simulink model "filter_bank"  (R2020b)
settings: Solver=FixedStepDiscrete  StartTime=0.0  StopTime=0.01  FixedStep=1.6276041666666666e-07  RelTol=1e-3
undefined symbols (not defined in the file or in its folder): mp
libraries: hdlsllib x2, simulink x1
settings Model: DataTypeOverride=Off  Creator=Ross  LastModifiedBy=conno
settings DataIOCC: SaveOutput=off  SaveTime=off  ReturnWorkspaceOutputs=off
settings OptimizationCC: BlockReduction=off  ConditionallyExecuteInputs=off  DefaultParameterBehavior=Inlined
settings DebuggingCC: ReadBeforeWriteMsg=DisableAll  WriteAfterWriteMsg=DisableAll  WriteAfterReadMsg=DisableAll  AlgebraicLoopMsg=error  MultiTaskDSMMsg=none  SingleTaskRateTransMsg=error  PregeneratedLibrarySubsystemCodeDiagnostic=none  ArithmeticOperatorsInVariantConditions=warning
settings HardwareCC: ProdBitPerPointer=32  ProdBitPerSizeT=32  ProdBitPerPtrDiffT=32  ProdLargestAtomicFloat=None  ProdIntDivRoundTo=Undefined  ProdEndianess=Unspecified  ProdWordSize=32  ProdHWDeviceType=ASIC/FPGA->ASIC/FPGA  TargetBitPerPointer=64  TargetBitPerSizeT=64  TargetBitPerPtrDiffT=64  TargetLongLongMode=on  TargetIntDivRoundTo=Zero  TargetEndianess=LittleEndian  TargetWordSize=64  TargetHWDeviceType=Custom Processor->MATLAB Host Computer  ProdEqTarget=off
settings ModelReferenceCC: UpdateModelReferenceTargets=IfOutOfDate
settings SFSimCC: SFSimEcho=off  SimUseLocalCustomCode=off  CustomCodeUndefinedFunction=UseInterfaceOnly
settings RTWCC: RTWUseLocalCustomCode=off

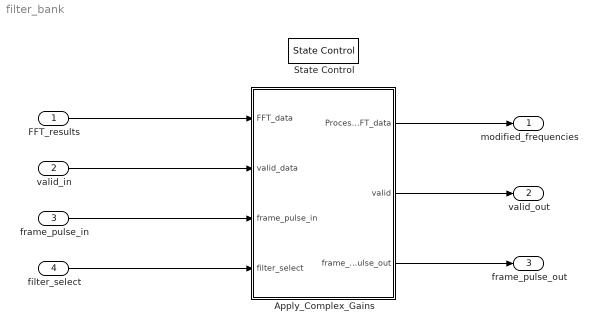
== system filter_bank ==
  FFT_results : Inport  OutDataTypeStr=fixdt(1,31,23)  PortDimensions=1  SampleTime=[1.6276041666666666e-07,0]
      settings: SignalType=complex
  valid_in : Inport  Port=2  OutDataTypeStr=boolean  PortDimensions=1  SampleTime=[1.6276041666666666e-07,0]
  frame_pulse_in : Inport  Port=3  OutDataTypeStr=boolean  PortDimensions=1  SampleTime=[1.6276041666666666e-07,0]
  filter_select : Inport  Port=4  OutDataTypeStr=fixdt(0,2,0)  PortDimensions=1  SampleTime=[1.6276041666666666e-07,0]
  Apply_Complex_Gains : Subsystem
  State Control : StateControl  StateControl=Synchronous
  modified_frequencies : Outport  PortDimensions=1  SampleTime=[1.6276041666666666e-07,0]  VectorParamsAs1DForOutWhenUnconnected=off
      settings: SignalType=complex
  valid_out : Outport  Port=2  OutDataTypeStr=boolean  PortDimensions=1  SampleTime=[1.6276041666666666e-07,0]  VectorParamsAs1DForOutWhenUnconnected=off
  frame_pulse_out : Outport  Port=3  OutDataTypeStr=boolean  PortDimensions=1  SampleTime=[1.6276041666666666e-07,0]
  wires:
  FFT_results/1 -> Apply_Complex_Gains/1(FFT_data)
  valid_in/1 -> Apply_Complex_Gains/2(valid_data)
  frame_pulse_in/1 -> Apply_Complex_Gains/3(frame_pulse_in)
  Apply_Complex_Gains/1(Processed_FFT_data) -> modified_frequencies/1
  Apply_Complex_Gains/2(valid) -> valid_out/1
  Apply_Complex_Gains/3(frame_pulse_out) -> frame_pulse_out/1
  filter_select/1 -> Apply_Complex_Gains/4(filter_select)

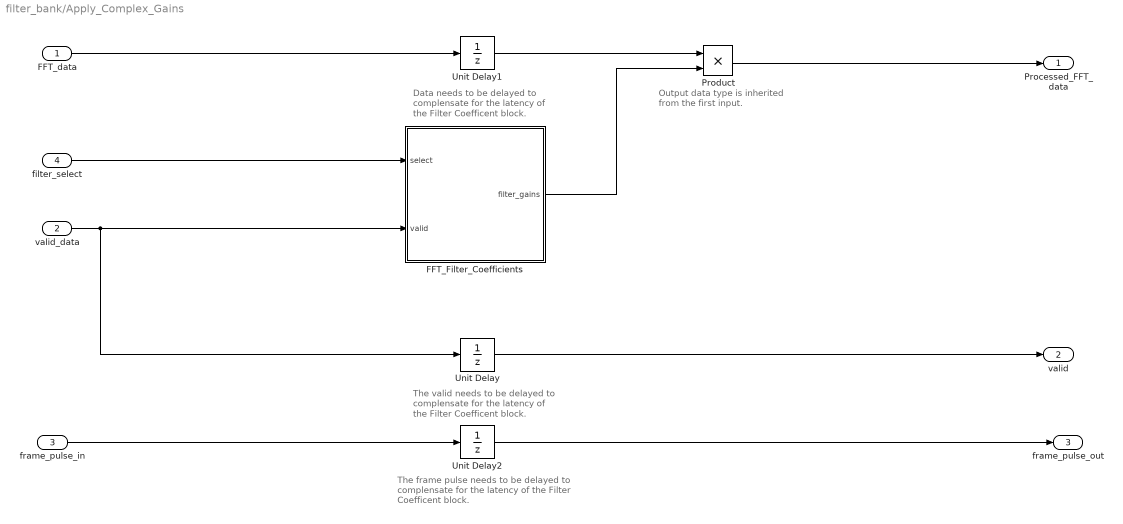
== system filter_bank/Apply_Complex_Gains ==
  note: Data needs to be delayed
      | to complensate for the latency
      | of the Filter Coefficent block.
  note: The valid needs to be delayed
      | to complensate for the latency
      | of the Filter Coefficent block.
  note: The frame pulse needs to be delayed
      | to complensate for the latency
      | of the Filter Coefficent block.
  note: Output data type is inherited
      | from the first input.
  FFT_data : Inport
  valid_data : Inport  Port=2
  frame_pulse_in : Inport  Port=3
  filter_select : Inport  Port=4
  FFT_Filter_Coefficients : Subsystem
  Product : Product  OutDataTypeStr=Inherit: Same as first input
  Unit Delay : UnitDelay  SampleTime=-1  HasFrameUpgradeWarning=on
  Unit Delay1 : UnitDelay  SampleTime=-1  HasFrameUpgradeWarning=on
  Unit Delay2 : UnitDelay  SampleTime=-1  HasFrameUpgradeWarning=on
  Processed_FFT_data : Outport
  valid : Outport  Port=2
  frame_pulse_out : Outport  Port=3
  wires:
  Unit Delay1/1 -> Product/1
  Unit Delay/1 -> valid/1
  Product/1 -> Processed_FFT_data/1
  FFT_Filter_Coefficients/1(filter_gains) -> Product/2
  filter_select/1 -> FFT_Filter_Coefficients/1(select)
  Unit Delay2/1 -> frame_pulse_out/1
  frame_pulse_in/1 -> Unit Delay2/1
  FFT_data/1 -> Unit Delay1/1
  valid_data/1 -> FFT_Filter_Coefficients/2(valid), Unit Delay/1

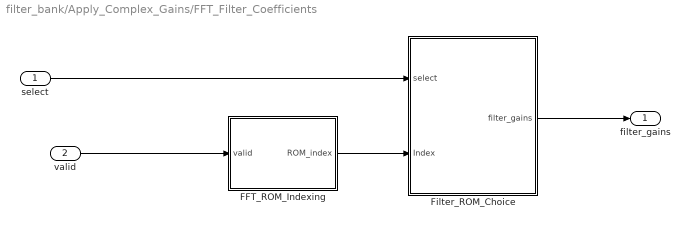
== system filter_bank/Apply_Complex_Gains/FFT_Filter_Coefficients ==
  select : Inport
  valid : Inport  Port=2
  FFT_ROM_Indexing : Subsystem
  Filter_ROM_Choice : Subsystem
  filter_gains : Outport
  wires:
  Filter_ROM_Choice/1(filter_gains) -> filter_gains/1
  select/1 -> Filter_ROM_Choice/1(select)
  valid/1 -> FFT_ROM_Indexing/1(valid)
  FFT_ROM_Indexing/1(ROM_index) -> Filter_ROM_Choice/2(Index)

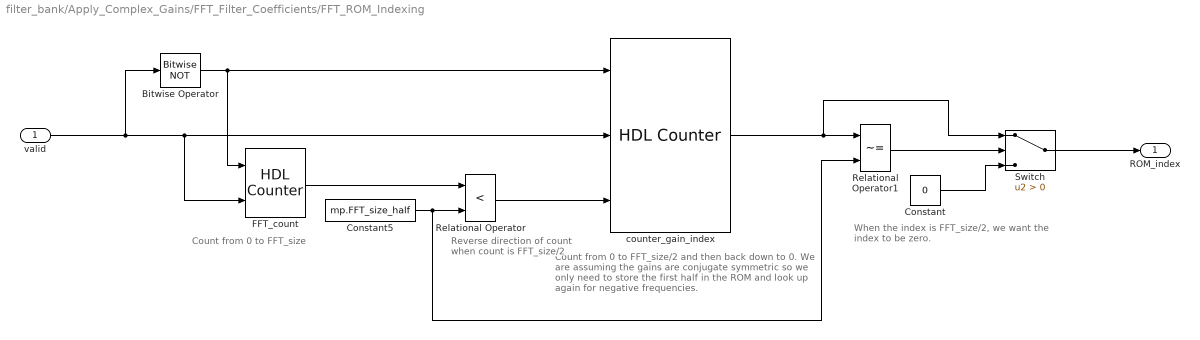
== system filter_bank/Apply_Complex_Gains/FFT_Filter_Coefficients/FFT_ROM_Indexing ==
  note: Count from 0 to FFT_size/2 and then back down to 0.
      | We are assuming the gains are conjugate symmetric
      | so we only need to store the first half in the ROM
      | and look up again for negative frequencies.
  note: Reverse direction of
      | count when count
      | is FFT_size/2
  note: Count from 0 to FFT_size
  note: When the index is FFT_size/2, we want the
      | index to be zero.
  valid : Inport
  Bitwise Operator : simulink/Logic and Bit Operations/Bitwise Operator  logicop=NOT  UseBitMask=off  BitMask=bin2dec('11011001')  BitMaskRealWorld=Stored Integer
  Constant : Constant  Value=0  OutDataTypeStr=fixdt(0,mp.FFT_size_Nbits,0)  SampleTime=mp.Ts/mp.SysRate_Upsample_Factor
  Constant5 : Constant  Value=mp.FFT_size_half  OutDataTypeStr=fixdt(0,mp.FFT_size_Nbits,0)  SampleTime=mp.Ts/mp.SysRate_Upsample_Factor
  FFT_count : hdlsllib/Sources/HDL Counter  CountType=Free running  CountInit=0  CountStep=1  CountMax=25  CountFromType=Initial value  CountFrom=0  CountResetPort=on  CountLoadPort=off  CountEnbPort=on  CountDirPort=off  CountDataType=Unsigned  CountWordLen=mp.FFT_size_Nbits  CountFracLen=0  CountSampTime=1
  Relational Operator : RelationalOperator  Operator=<  OutDataTypeStr=boolean  ZeroCross=off  RndMeth=Nearest
  Relational Operator1 : RelationalOperator  Operator=~=  OutDataTypeStr=boolean  ZeroCross=off  RndMeth=Nearest
  Switch : Switch  Criteria=u2 > Threshold
  counter_gain_index : hdlsllib/Sources/HDL Counter  CountType=Free running  CountInit=0  CountStep=1  CountMax=25  CountFromType=Initial value  CountFrom=0  CountResetPort=on  CountLoadPort=off  CountEnbPort=on  CountDirPort=on  CountDataType=Unsigned  CountWordLen=mp.FFT_size_Nbits  CountFracLen=0  CountSampTime=1
  ROM_index : Outport
  wires:
  Switch/1 -> ROM_index/1
  Constant/1 -> Switch/3
  counter_gain_index/1 -> Relational Operator1/1, Switch/1
  Constant5/1 -> Relational Operator/2, Relational Operator1/2
  valid/1 -> Bitwise Operator/1, counter_gain_index/2, FFT_count/2
  FFT_count/1 -> Relational Operator/1
  Relational Operator1/1 -> Switch/2
  Bitwise Operator/1 -> counter_gain_index/1, FFT_count/1
  Relational Operator/1 -> counter_gain_index/3

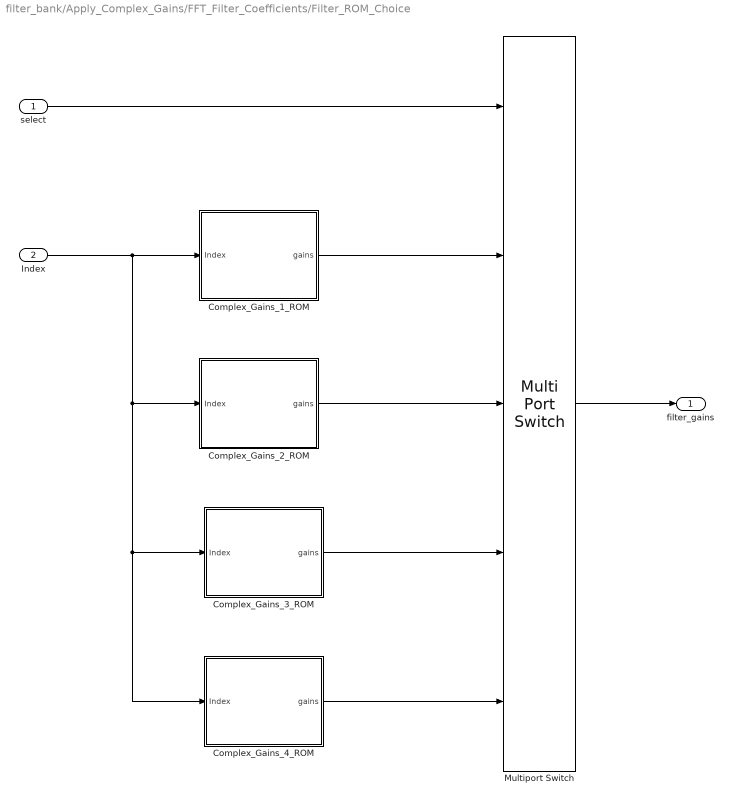
== system filter_bank/Apply_Complex_Gains/FFT_Filter_Coefficients/Filter_ROM_Choice ==
  select : Inport
  Index : Inport  Port=2
  Complex_Gains_1_ROM : Subsystem
  Complex_Gains_2_ROM : Subsystem
  Complex_Gains_3_ROM : Subsystem
  Complex_Gains_4_ROM : Subsystem
  Multiport Switch : MultiPortSwitch  DataPortOrder=Zero-based contiguous  Inputs=4  zeroidx=on
  filter_gains : Outport
  wires:
  Complex_Gains_3_ROM/1(gains) -> Multiport Switch/4
  select/1 -> Multiport Switch/1
  Complex_Gains_2_ROM/1(gains) -> Multiport Switch/3
  Complex_Gains_1_ROM/1(gains) -> Multiport Switch/2
  Complex_Gains_4_ROM/1(gains) -> Multiport Switch/5
  Index/1 -> Complex_Gains_4_ROM/1(Index), Complex_Gains_3_ROM/1(Index), Complex_Gains_2_ROM/1(Index), Complex_Gains_1_ROM/1(Index)
  Multiport Switch/1 -> filter_gains/1

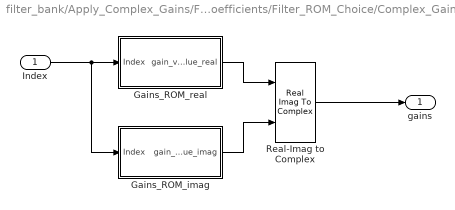
== system filter_bank/Apply_Complex_Gains/FFT_Filter_Coefficients/Filter_ROM_Choice/Complex_Gains_1_ROM ==
  Index : Inport
  Gains_ROM_imag : Subsystem
  Gains_ROM_real : Subsystem
  Real-Imag to Complex : RealImagToComplex
  gains : Outport
  wires:
  Real-Imag to Complex/1 -> gains/1
  Gains_ROM_real/1(gain_value_real) -> Real-Imag to Complex/1
  Index/1 -> Gains_ROM_real/1(Index), Gains_ROM_imag/1(Index)
  Gains_ROM_imag/1(gain_value_imag) -> Real-Imag to Complex/2

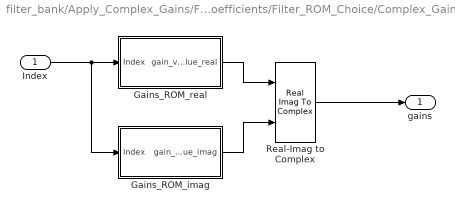
== system filter_bank/Apply_Complex_Gains/FFT_Filter_Coefficients/Filter_ROM_Choice/Complex_Gains_2_ROM ==
  Index : Inport
  Gains_ROM_imag : Subsystem
  Gains_ROM_real : Subsystem
  Real-Imag to Complex : RealImagToComplex
  gains : Outport
  wires:
  Real-Imag to Complex/1 -> gains/1
  Gains_ROM_real/1(gain_value_real) -> Real-Imag to Complex/1
  Index/1 -> Gains_ROM_real/1(Index), Gains_ROM_imag/1(Index)
  Gains_ROM_imag/1(gain_value_imag) -> Real-Imag to Complex/2

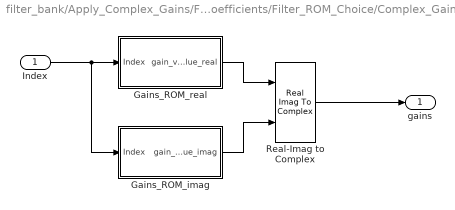
== system filter_bank/Apply_Complex_Gains/FFT_Filter_Coefficients/Filter_ROM_Choice/Complex_Gains_3_ROM ==
  Index : Inport
  Gains_ROM_imag : Subsystem
  Gains_ROM_real : Subsystem
  Real-Imag to Complex : RealImagToComplex
  gains : Outport
  wires:
  Real-Imag to Complex/1 -> gains/1
  Gains_ROM_real/1(gain_value_real) -> Real-Imag to Complex/1
  Index/1 -> Gains_ROM_real/1(Index), Gains_ROM_imag/1(Index)
  Gains_ROM_imag/1(gain_value_imag) -> Real-Imag to Complex/2

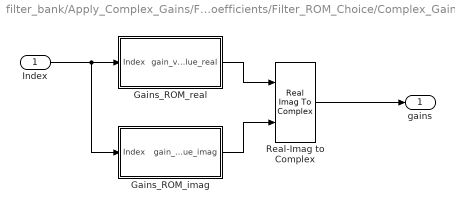
== system filter_bank/Apply_Complex_Gains/FFT_Filter_Coefficients/Filter_ROM_Choice/Complex_Gains_4_ROM ==
  Index : Inport
  Gains_ROM_imag : Subsystem
  Gains_ROM_real : Subsystem
  Real-Imag to Complex : RealImagToComplex
  gains : Outport
  wires:
  Real-Imag to Complex/1 -> gains/1
  Gains_ROM_real/1(gain_value_real) -> Real-Imag to Complex/1
  Index/1 -> Gains_ROM_real/1(Index), Gains_ROM_imag/1(Index)
  Gains_ROM_imag/1(gain_value_imag) -> Real-Imag to Complex/2

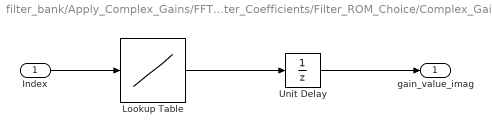
== system filter_bank/Apply_Complex_Gains/FFT_Filter_Coefficients/Filter_ROM_Choice/Complex_Gains_1_ROM/Gains_ROM_imag ==
  Index : Inport
  Lookup Table : Lookup_n-D  NumberOfTableDimensions=1  BreakpointsForDimension1=[0:mp.FFT_size_half-1]  IndexSearchMethod=Evenly spaced points  Table=mp.fft_gains_1_imag  InterpMethod=Flat  ExtrapMethod=Clip  DiagnosticForOutOfRangeInput=Error  UseLastTableValue=on  OutDataTypeStr=fixdt(1,mp.W_bits,mp.F_bits)  RndMeth=Simplest  InputSameDT=on
  Unit Delay : UnitDelay  SampleTime=-1  HasFrameUpgradeWarning=on
  gain_value_imag : Outport  VectorParamsAs1DForOutWhenUnconnected=off
  wires:
  Lookup Table/1 -> Unit Delay/1
  Index/1 -> Lookup Table/1
  Unit Delay/1 -> gain_value_imag/1

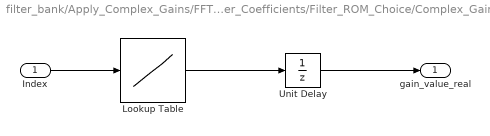
== system filter_bank/Apply_Complex_Gains/FFT_Filter_Coefficients/Filter_ROM_Choice/Complex_Gains_1_ROM/Gains_ROM_real ==
  Index : Inport
  Lookup Table : Lookup_n-D  NumberOfTableDimensions=1  BreakpointsForDimension1=[0:mp.FFT_size_half-1]  IndexSearchMethod=Evenly spaced points  Table=mp.fft_gains_1_real  InterpMethod=Flat  ExtrapMethod=Clip  DiagnosticForOutOfRangeInput=Error  UseLastTableValue=on  OutDataTypeStr=fixdt(1,mp.W_bits,mp.F_bits)  RndMeth=Simplest  InputSameDT=on
  Unit Delay : UnitDelay  SampleTime=-1  HasFrameUpgradeWarning=on
  gain_value_real : Outport  VectorParamsAs1DForOutWhenUnconnected=off
  wires:
  Lookup Table/1 -> Unit Delay/1
  Index/1 -> Lookup Table/1
  Unit Delay/1 -> gain_value_real/1

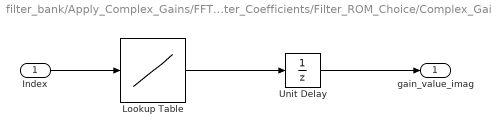
== system filter_bank/Apply_Complex_Gains/FFT_Filter_Coefficients/Filter_ROM_Choice/Complex_Gains_2_ROM/Gains_ROM_imag ==
  Index : Inport
  Lookup Table : Lookup_n-D  NumberOfTableDimensions=1  BreakpointsForDimension1=[0:mp.FFT_size_half-1]  IndexSearchMethod=Evenly spaced points  Table=mp.fft_gains_2_imag  InterpMethod=Flat  ExtrapMethod=Clip  DiagnosticForOutOfRangeInput=Error  UseLastTableValue=on  OutDataTypeStr=fixdt(1,mp.W_bits,mp.F_bits)  RndMeth=Simplest  InputSameDT=on
  Unit Delay : UnitDelay  SampleTime=-1  HasFrameUpgradeWarning=on
  gain_value_imag : Outport  VectorParamsAs1DForOutWhenUnconnected=off
  wires:
  Lookup Table/1 -> Unit Delay/1
  Index/1 -> Lookup Table/1
  Unit Delay/1 -> gain_value_imag/1

== system filter_bank/Apply_Complex_Gains/FFT_Filter_Coefficients/Filter_ROM_Choice/Complex_Gains_2_ROM/Gains_ROM_real ==
  Index : Inport
  Lookup Table : Lookup_n-D  NumberOfTableDimensions=1  BreakpointsForDimension1=[0:mp.FFT_size_half-1]  IndexSearchMethod=Evenly spaced points  Table=mp.fft_gains_2_real  InterpMethod=Flat  ExtrapMethod=Clip  DiagnosticForOutOfRangeInput=Error  UseLastTableValue=on  OutDataTypeStr=fixdt(1,mp.W_bits,mp.F_bits)  RndMeth=Simplest  InputSameDT=on
  Unit Delay : UnitDelay  SampleTime=-1  HasFrameUpgradeWarning=on
  gain_value_real : Outport  VectorParamsAs1DForOutWhenUnconnected=off
  wires:
  Lookup Table/1 -> Unit Delay/1
  Index/1 -> Lookup Table/1
  Unit Delay/1 -> gain_value_real/1

== system filter_bank/Apply_Complex_Gains/FFT_Filter_Coefficients/Filter_ROM_Choice/Complex_Gains_3_ROM/Gains_ROM_imag ==
  Index : Inport
  Lookup Table : Lookup_n-D  NumberOfTableDimensions=1  BreakpointsForDimension1=[0:mp.FFT_size_half-1]  IndexSearchMethod=Evenly spaced points  Table=mp.fft_gains_3_imag  InterpMethod=Flat  ExtrapMethod=Clip  DiagnosticForOutOfRangeInput=Error  UseLastTableValue=on  OutDataTypeStr=fixdt(1,mp.W_bits,mp.F_bits)  RndMeth=Simplest  InputSameDT=on
  Unit Delay : UnitDelay  SampleTime=-1  HasFrameUpgradeWarning=on
  gain_value_imag : Outport  VectorParamsAs1DForOutWhenUnconnected=off
  wires:
  Lookup Table/1 -> Unit Delay/1
  Index/1 -> Lookup Table/1
  Unit Delay/1 -> gain_value_imag/1

== system filter_bank/Apply_Complex_Gains/FFT_Filter_Coefficients/Filter_ROM_Choice/Complex_Gains_3_ROM/Gains_ROM_real ==
  Index : Inport
  Lookup Table : Lookup_n-D  NumberOfTableDimensions=1  BreakpointsForDimension1=[0:mp.FFT_size_half-1]  IndexSearchMethod=Evenly spaced points  Table=mp.fft_gains_3_real  InterpMethod=Flat  ExtrapMethod=Clip  DiagnosticForOutOfRangeInput=Error  UseLastTableValue=on  OutDataTypeStr=fixdt(1,mp.W_bits,mp.F_bits)  RndMeth=Simplest  InputSameDT=on
  Unit Delay : UnitDelay  SampleTime=-1  HasFrameUpgradeWarning=on
  gain_value_real : Outport  VectorParamsAs1DForOutWhenUnconnected=off
  wires:
  Lookup Table/1 -> Unit Delay/1
  Index/1 -> Lookup Table/1
  Unit Delay/1 -> gain_value_real/1

== system filter_bank/Apply_Complex_Gains/FFT_Filter_Coefficients/Filter_ROM_Choice/Complex_Gains_4_ROM/Gains_ROM_imag ==
  Index : Inport
  Lookup Table : Lookup_n-D  NumberOfTableDimensions=1  BreakpointsForDimension1=[0:mp.FFT_size_half-1]  IndexSearchMethod=Evenly spaced points  Table=mp.fft_gains_4_imag  InterpMethod=Flat  ExtrapMethod=Clip  DiagnosticForOutOfRangeInput=Error  UseLastTableValue=on  OutDataTypeStr=fixdt(1,mp.W_bits,mp.F_bits)  RndMeth=Simplest  InputSameDT=on
  Unit Delay : UnitDelay  SampleTime=-1  HasFrameUpgradeWarning=on
  gain_value_imag : Outport  VectorParamsAs1DForOutWhenUnconnected=off
  wires:
  Lookup Table/1 -> Unit Delay/1
  Index/1 -> Lookup Table/1
  Unit Delay/1 -> gain_value_imag/1

== system filter_bank/Apply_Complex_Gains/FFT_Filter_Coefficients/Filter_ROM_Choice/Complex_Gains_4_ROM/Gains_ROM_real ==
  Index : Inport
  Lookup Table : Lookup_n-D  NumberOfTableDimensions=1  BreakpointsForDimension1=[0:mp.FFT_size_half-1]  IndexSearchMethod=Evenly spaced points  Table=mp.fft_gains_4_real  InterpMethod=Flat  ExtrapMethod=Clip  DiagnosticForOutOfRangeInput=Error  UseLastTableValue=on  OutDataTypeStr=fixdt(1,mp.W_bits,mp.F_bits)  RndMeth=Simplest  InputSameDT=on
  Unit Delay : UnitDelay  SampleTime=-1  HasFrameUpgradeWarning=on
  gain_value_real : Outport  VectorParamsAs1DForOutWhenUnconnected=off
  wires:
  Lookup Table/1 -> Unit Delay/1
  Index/1 -> Lookup Table/1
  Unit Delay/1 -> gain_value_real/1
